simulink model "userGuide_1_understanding_2_littleTutorial"  (R2014b)
settings: Solver=ode15s  StartTime=0.0  StopTime=10.0  RelTol=1e-3
libraries: nesl_utility x4, FINALFluidHeliumLibrary x4, fluidHelium_lib x2
settings Model: Creator=vassalad  LastModifiedBy=vassalad
settings SimscapeCC: SimscapeLogType=all

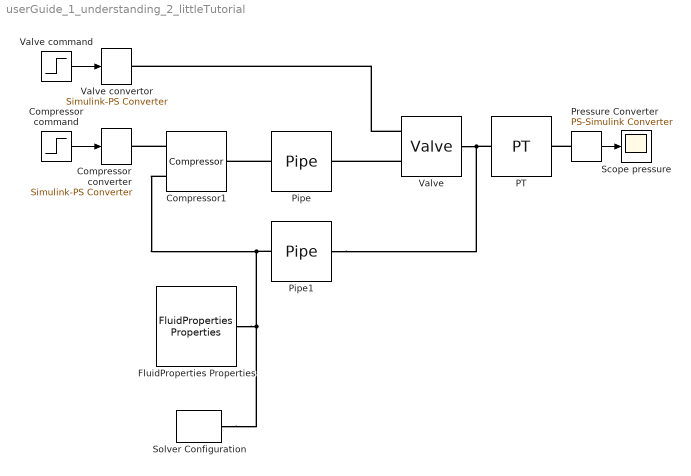
== system userGuide_1_understanding_2_littleTutorial ==
  Compressor command : Step  Time=5  Before=5  After=5  SampleTime=0
  Compressor converter : nesl_utility/Simulink-PS Converter  PhysicalDomain=network_engine_domain  SubClassName=ps_input  LeftPortType=input  RightPortType=output  PseudoPeriodic=off  Frequencies=[]  NoiseDistribution=none  NoiseParameters=[]  Unit=1  AffineConversion=off  InputFiltering=off  SimscapeFilterOrder=1  InputFilterTimeConstant=0.001  UdotUserProvided=1
  Compressor1 : FINALFluidHeliumLibrary/Elements/Compressor  Kc=Kc kg/rad/bar  ControlInputMin=ControlInputMin rad/s  ControlInputMax=ControlInputMax rad/s  T_specify=off  T_priority=High  T=0 K  mask(Compressor){Kc=0.0014, Kc_unit=kg/rad/bar, ControlInputMin=0.001, ControlInputMin_unit=rad/s, ControlInputMax=10, ControlInputMax_unit=rad/s}
      mask prompts: Kc "Compressor constant"; ControlInputMin "Minimum allowed compressor control"; ControlInputMax "Maximum allowed compressor control"
      mask help:
      | Compressor
      |
      |     This component is an isothermal screw compressor. This component is imposing
      |     both inlet and outlet flow rate, as well as output temperature.
      |
      |     To ensure compilation, you must connect the inlet
      |     port to a component that impose both pressure and temperature (such a pipe outlet).
      |     The outlet port must be connected to a component that impose pressure (such a pipe inlet)
      |
      |     The parameter Kc must be positive
      mask Help: eval('open(''P:/_donnees PI/PI02/Adrien/Matlab/Simscape/FluidHeliumV4.3.3/FluidHeliumMPH/Help/blocks_1_elements_1_compressor.html'')');
      mask TypeOptions Kc: Kc
      mask TypeOptions Kc_unit: Kc_unit
      mask TypeOptions ControlInputMin: ControlInputMin
      mask TypeOptions ControlInputMin_unit: ControlInputMin_unit
      mask TypeOptions ControlInputMax: ControlInputMax
      mask TypeOptions ControlInputMax_unit: ControlInputMax_unit
  FluidProperties Properties : fluidHelium_lib/Utilities/FluidProperties Properties  P_min=0.01 bar  T_min=1 K  T_max=100 K  P_max=50 bar  Mol=4.0026 * 10 ^ (- 3) kg/mol
  PT : fluidHelium_lib/Sensors/PT
  Pipe : FINALFluidHeliumLibrary/Elements/Pipe  Vol=Vol m^3  P0=P0 bar  T0=T0 K  Ideal=Ideal  rho_specify=off  rho_priority=High  rho=0 kg/m^3  rho_p_specify=off  rho_p_priority=High  rho_p=0 kg/m^3/s  u_specify=off  u_priority=High  u=0 J/kg  P_specify=off  P_priority=High  P=0 bar  T_specify=off  T_priority=High  T=0 K  mask(Pipe){Vol=0.01, Vol_unit=m^3, Ideal=1, Ideal_unit=1, P0=16, P0_unit=bar, T0=90, T0_unit=K}
      mask prompts: Vol "Volume of the pipe"; Ideal "Ideal 1/0"; P0 "Initial pressure of the pipe"; T0 "Initial temperature of the pipe"
      mask help:
      | Pipe
      |
      |     This component is a 0D pipe. It is different than a simple port connection
      |     because it impose a variable pressure on both inlet and outlet ports.
      |     The temperature is also imposed on the outlet port.
      |
      |     To ensure compilation, the 0D pipe inlet port must be connected to a
      |     component port that impose both temperature and flow rate (such as a
      |     compressor outlet or a valve outlet). The 0D pipe outlet port must be
      |     connected to a component port that impose the flow rate (such as a
      |     compressor inlet or a valve inlet).
      |
      |     If you want to use an ideal pipe (differentiation of P wrt time)
      |     the parameter 'Ideal' must be set to 1. Otherwise, a non-Ideal pipe
      |     (differentiation of rho and u wrt time) will be used
      |
      |     The parameters Vol and initial conditions P0 and T0 must be positive
      mask TypeOptions Vol: Vol
      mask TypeOptions Vol_unit: Vol_unit
      mask TypeOptions Ideal: Ideal
      mask TypeOptions Ideal_unit: Ideal_unit
      mask TypeOptions P0: P0
      mask TypeOptions P0_unit: P0_unit
      mask TypeOptions T0: T0
      mask TypeOptions T0_unit: T0_unit
  Pipe1 : FINALFluidHeliumLibrary/Elements/Pipe  Vol=Vol m^3  P0=P0 bar  T0=T0 K  Ideal=Ideal  rho_specify=off  rho_priority=High  rho=0 kg/m^3  rho_p_specify=off  rho_p_priority=High  rho_p=0 kg/m^3/s  u_specify=off  u_priority=High  u=0 J/kg  P_specify=off  P_priority=High  P=0 bar  T_specify=off  T_priority=High  T=0 K  mask(Pipe){Vol=0.01, Vol_unit=m^3, Ideal=1, Ideal_unit=1, P0=1.05, P0_unit=bar, T0=70, T0_unit=K}
      mask prompts: Vol "Volume of the pipe"; Ideal "Ideal 1/0"; P0 "Initial pressure of the pipe"; T0 "Initial temperature of the pipe"
      mask help:
      | Pipe
      |
      |     This component is a 0D pipe. It is different than a simple port connection
      |     because it impose a variable pressure on both inlet and outlet ports.
      |     The temperature is also imposed on the outlet port.
      |
      |     To ensure compilation, the 0D pipe inlet port must be connected to a
      |     component port that impose both temperature and flow rate (such as a
      |     compressor outlet or a valve outlet). The 0D pipe outlet port must be
      |     connected to a component port that impose the flow rate (such as a
      |     compressor inlet or a valve inlet).
      |
      |     If you want to use an ideal pipe (differentiation of P wrt time)
      |     the parameter 'Ideal' must be set to 1. Otherwise, a non-Ideal pipe
      |     (differentiation of rho and u wrt time) will be used
      |
      |     The parameters Vol and initial conditions P0 and T0 must be positive
      mask TypeOptions Vol: Vol
      mask TypeOptions Vol_unit: Vol_unit
      mask TypeOptions Ideal: Ideal
      mask TypeOptions Ideal_unit: Ideal_unit
      mask TypeOptions P0: P0
      mask TypeOptions P0_unit: P0_unit
      mask TypeOptions T0: T0
      mask TypeOptions T0_unit: T0_unit
  Pressure Converter : nesl_utility/PS-Simulink Converter  PhysicalDomain=network_engine_domain  SubClassName=ps_output  LeftPortType=input  RightPortType=output  PseudoPeriodic=off  Frequencies=[]  Unit=1  AffineConversion=off
  Scope pressure : Scope
      settings: YMin=0  YMax=1
  Solver Configuration : nesl_utility/Solver Configuration  PhysicalDomain=network_engine_domain  SubClassName=solver  LeftPortType=input  RightPortType=generic  Accelerate=off  Tones=[]  Harmonics=[]  SimulateNoise=off  Profile=off  UseLocalSampling=off  EnableSwitchedLinearOptims=on  FrequencyDomain=off  UseCCode=off  RelTol=0.001  AbsTol=1e-06  MinStep=1e-09  ToWorkspace=off  DoDC=off  ResidualTolerance=1e-09  UseLocalSolver=off  LocalSolverChoice=NE_BACKWARD_EULER_ADVANCER  LocalSolverSampleTime=0.001  DoFixedCost=off  MaxNonlinIter=3  MaxModeIter=2  LinearAlgebra=Sparse  DelaysMemoryBudget=1024  AutomaticFiltering=on  FilteringTimeConstant=0.001
  Valve : FINALFluidHeliumLibrary/Elements/Valve  CVmax=CVmax  ControlInputMin=ControlInputMin  ControlInputMax=ControlInputMax  Xt=Xt  Rv=Rv  K=2.4e-5 m^1.50000*kg^0.50000/s/bar^0.50000  Cmd_specify=off  Cmd_priority=High  Cmd=0  gamma_specify=off  gamma_priority=High  gamma=0  rho_specify=off  rho_priority=High  rho=0 kg/m^3  Xc_specify=off  Xc_priority=High  Xc=0  X_specify=off  X_priority=High  X=0  Y_specify=off  Y_priority=High  Y=0  CV_specify=off  CV_priority=High  CV=0  mask(Valve){CVmax=3.2, CVmax_unit=1, Xt=0.86, Xt_unit=1, Rv=10, Rv_unit=1, ControlInputMin=0, ControlInputMin_unit=1, ControlInputMax=100, ControlInputMax_unit=1}
      mask prompts: CVmax "Valve constant"; Xt "Xt valve constructor constant"; Rv "Rv valve constructor constant"; ControlInputMin "Minimum allowed for valve control"; ControlInputMax "Maximum allowed for valve control"
      mask help:
      | Valve
      |
      |     This component is a valve, it's allowed you to regulate pressure and mass flow
      |
      |     For a good use of this component you must respect the following point :
      |
      |     The CVmax, Xt and Rv parameters must be greater than 0
      |
      |     The opening of the valve ( C ) must be comprised between CMin and CMax percent
      |
      |      Connect to the input of the valve a component that imposed the temperature and pressure
      |     (not the flow rate)
      |
      |      Connect to the output of the valve a component that imposed the pressure
      |     (not the flow rate neither the temperature)
      mask TypeOptions CVmax: CVmax
      mask TypeOptions CVmax_unit: CVmax_unit
      mask TypeOptions Xt: Xt
      mask TypeOptions Xt_unit: Xt_unit
      mask TypeOptions Rv: Rv
      mask TypeOptions Rv_unit: Rv_unit
      mask TypeOptions ControlInputMin: ControlInputMin
      mask TypeOptions ControlInputMin_unit: ControlInputMin_unit
      mask TypeOptions ControlInputMax: ControlInputMax
      mask TypeOptions ControlInputMax_unit: ControlInputMax_unit
  Valve command : Step  Before=50  After=50  SampleTime=0
  Valve convertor : nesl_utility/Simulink-PS Converter  PhysicalDomain=network_engine_domain  SubClassName=ps_input  LeftPortType=input  RightPortType=output  PseudoPeriodic=off  Frequencies=[]  NoiseDistribution=none  NoiseParameters=[]  Unit=1  AffineConversion=off  InputFiltering=off  SimscapeFilterOrder=1  InputFilterTimeConstant=0.001  UdotUserProvided=1
  wires:
  Compressor command/1 -> Compressor converter/1
  Valve command/1 -> Valve convertor/1
  Pressure Converter/1 -> Scope pressure/1
  connections:
  Pipe/LConn1 -- Compressor1/RConn1
  Valve/LConn2 -- Pipe/RConn1
  PT/LConn1 -- Valve/RConn1 -- Pipe1/LConn1
  FluidProperties Properties/RConn1 -- Solver Configuration/RConn1 -- Pipe1/RConn1 -- Compressor1/LConn2
  Compressor1/LConn1 -- Compressor converter/RConn1
  Valve/LConn1 -- Valve convertor/RConn1
  Pressure Converter/LConn1 -- PT/RConn1
